simulink model "pr735_DDC_demodulation"  (R2018b)
settings: Solver=VariableStepAuto  StartTime=0.0  StopTime=2048/fs  RelTol=1e-3
PreLoadFcn:
  | fs=1e8;
  | pr731_DUC_setup
  | pr734_DDC_setup;
  | fc=40e6;
undefined symbols (not defined in the file or in its folder): CFIR, CIC, DCIC, designMultirateFIR, RRC
libraries: dspmlti4 x12, commdigbbndpm3 x2, commrandsrc3 x1
settings Model: Creator=Григорий Фокин  LastModifiedBy=Григорий Фокин
settings DataIOCC: SaveFormat=Array  SaveOutput=off  SignalLogging=off  SaveTime=off
settings DebuggingCC: AlgebraicLoopMsg=error
settings HardwareCC: ProdBitPerPointer=32  ProdBitPerSizeT=32  ProdBitPerPtrDiffT=32  ProdLargestAtomicFloat=None  ProdIntDivRoundTo=Undefined  ProdEndianess=Unspecified  ProdWordSize=32  ProdHWDeviceType=ASIC/FPGA->ASIC/FPGA  TargetBitPerPointer=64  TargetBitPerSizeT=64  TargetBitPerPtrDiffT=64  TargetLongLongMode=on  TargetIntDivRoundTo=Zero  TargetEndianess=LittleEndian  TargetWordSize=64  TargetHWDeviceType=Custom Processor->MATLAB Host Computer  ProdEqTarget=off

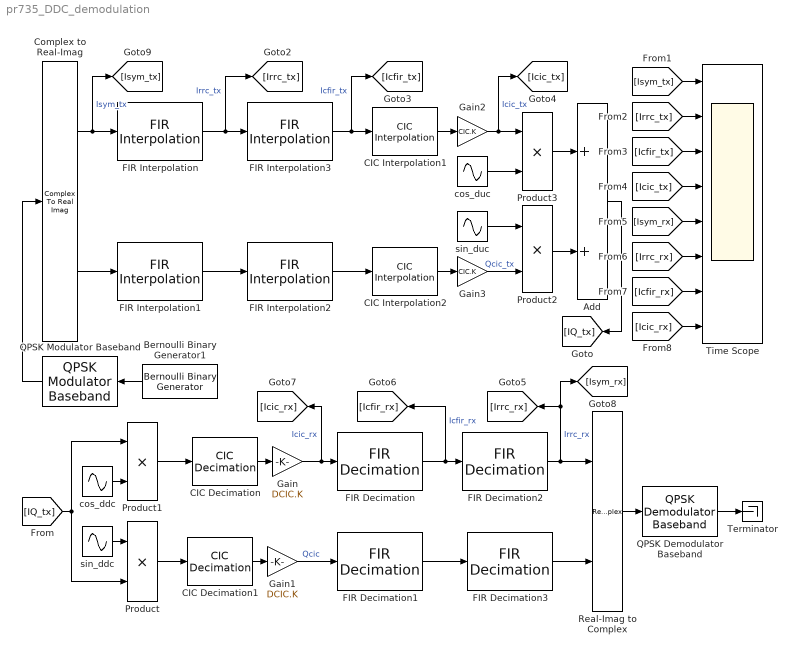
== system pr735_DDC_demodulation ==
  Add : Sum
  Bernoulli Binary Generator1 : commrandsrc3/Bernoulli Binary Generator  ProbabilityOfZero=0.5  SeedSource=Auto  Seed=0  SampleTime=(0.5*CIC.R*RRC.Lfactor*CFIR.Lfactor)/fs  SamplesPerFrame=2  OutputDataType=boolean  SimulateUsing=Interpreted execution
  CIC Decimation : dspmlti4/CIC Decimation  filtFrom=Multirate object in workspace  filtobj=hDCIC  ftype=Decimator  R=2  M=1  N=2  filterInternals=Full precision  BPS=[16 16 16 16]  FLPS=0  outputWordLength=32  outputFracLength=0  launchFVT=off  framing=Maintain input frame rate  RateOptions=Allow multirate processing
      settings: SourceProductName=DSP System Toolbox  SourceProductBaseCode=DS
  CIC Decimation1 : dspmlti4/CIC Decimation  filtFrom=Multirate object in workspace  filtobj=hDCIC  ftype=Decimator  R=2  M=1  N=2  filterInternals=Full precision  BPS=[16 16 16 16]  FLPS=0  outputWordLength=32  outputFracLength=0  launchFVT=off  framing=Maintain input frame rate  RateOptions=Allow multirate processing
      settings: SourceProductName=DSP System Toolbox  SourceProductBaseCode=DS
  CIC Interpolation1 : dspmlti4/CIC Interpolation  filtFrom=Multirate object in workspace  filtobj=hCIC  ftype=Interpolator  R=2  M=1  N=2  filterInternals=Full precision  BPS=[16 16 16 16]  FLPS=0  outputWordLength=32  outputFracLength=0  launchFVT=off  framing=Allow multirate processing  OutputFrames=off
      settings: SourceProductName=DSP System Toolbox  SourceProductBaseCode=DS
  CIC Interpolation2 : dspmlti4/CIC Interpolation  filtFrom=Multirate object in workspace  filtobj=hCIC  ftype=Interpolator  R=2  M=1  N=2  filterInternals=Full precision  BPS=[16 16 16 16]  FLPS=0  outputWordLength=32  outputFracLength=0  launchFVT=off  framing=Allow multirate processing  OutputFrames=off
      settings: SourceProductName=DSP System Toolbox  SourceProductBaseCode=DS
  Complex to Real-Imag : ComplexToRealImag
  FIR Decimation : dspmlti4/FIR Decimation  FilterSource=Filter object  h=designMultirateFIR(1,2)  D=2  filtStruct=Direct form  FilterObject=hDCFIR  framing=Enforce single-rate processing  inputOffset=0  outputBufInitCond=0  roundingMode=Floor  overflowMode=off  firstCoeffDataTypeStr=Inherit: Same word length as input  firstCoeffMin=[]  firstCoeffMax=[]  firstCoeffLastDataTypeStr=Inherit: Same word length as input  outputDataTypeStr=Inherit: Same as accumulator  outputMin=[]  outputMax=[]  outputLastDataTypeStr=Inherit: Same as accumulator
  FIR Decimation1 : dspmlti4/FIR Decimation  FilterSource=Filter object  h=designMultirateFIR(1,2)  D=2  filtStruct=Direct form  FilterObject=hDCFIR  framing=Enforce single-rate processing  inputOffset=0  outputBufInitCond=0  roundingMode=Floor  overflowMode=off  firstCoeffDataTypeStr=Inherit: Same word length as input  firstCoeffMin=[]  firstCoeffMax=[]  firstCoeffLastDataTypeStr=Inherit: Same word length as input  outputDataTypeStr=Inherit: Same as accumulator  outputMin=[]  outputMax=[]  outputLastDataTypeStr=Inherit: Same as accumulator
  FIR Decimation2 : dspmlti4/FIR Decimation  FilterSource=Filter object  h=designMultirateFIR(1,2)  D=2  filtStruct=Direct form  FilterObject=hDRRC  framing=Enforce single-rate processing  inputOffset=0  outputBufInitCond=0  roundingMode=Floor  overflowMode=off  firstCoeffDataTypeStr=Inherit: Same word length as input  firstCoeffMin=[]  firstCoeffMax=[]  firstCoeffLastDataTypeStr=Inherit: Same word length as input  outputDataTypeStr=Inherit: Same as accumulator  outputMin=[]  outputMax=[]  outputLastDataTypeStr=Inherit: Same as accumulator
  FIR Decimation3 : dspmlti4/FIR Decimation  FilterSource=Filter object  h=designMultirateFIR(1,2)  D=2  filtStruct=Direct form  FilterObject=hDRRC  framing=Enforce single-rate processing  inputOffset=0  outputBufInitCond=0  roundingMode=Floor  overflowMode=off  firstCoeffDataTypeStr=Inherit: Same word length as input  firstCoeffMin=[]  firstCoeffMax=[]  firstCoeffLastDataTypeStr=Inherit: Same word length as input  outputDataTypeStr=Inherit: Same as accumulator  outputMin=[]  outputMax=[]  outputLastDataTypeStr=Inherit: Same as accumulator
  FIR Interpolation : dspmlti4/FIR Interpolation  FilterSource=Filter object  h=designMultirateFIR(3,1)  L=3  FilterObject=hRRC  framing=Enforce single-rate processing  outputBufInitCond=0  roundingMode=Floor  overflowMode=off  firstCoeffDataTypeStr=Inherit: Same word length as input  firstCoeffMin=[]  firstCoeffMax=[]  firstCoeffLastDataTypeStr=Inherit: Same word length as input  outputDataTypeStr=Inherit: Same as accumulator  outputMin=[]  outputMax=[]  outputLastDataTypeStr=Inherit: Same as accumulator
      settings: SourceProductName=DSP System Toolbox
  FIR Interpolation1 : dspmlti4/FIR Interpolation  FilterSource=Filter object  h=designMultirateFIR(3,1)  L=3  FilterObject=hRRC  framing=Enforce single-rate processing  outputBufInitCond=0  roundingMode=Floor  overflowMode=off  firstCoeffDataTypeStr=Inherit: Same word length as input  firstCoeffMin=[]  firstCoeffMax=[]  firstCoeffLastDataTypeStr=Inherit: Same word length as input  outputDataTypeStr=Inherit: Same as accumulator  outputMin=[]  outputMax=[]  outputLastDataTypeStr=Inherit: Same as accumulator
      settings: SourceProductName=DSP System Toolbox
  FIR Interpolation2 : dspmlti4/FIR Interpolation  FilterSource=Filter object  h=designMultirateFIR(3,1)  L=3  FilterObject=hCFIR  framing=Enforce single-rate processing  outputBufInitCond=0  roundingMode=Floor  overflowMode=off  firstCoeffDataTypeStr=Inherit: Same word length as input  firstCoeffMin=[]  firstCoeffMax=[]  firstCoeffLastDataTypeStr=Inherit: Same word length as input  outputDataTypeStr=Inherit: Same as accumulator  outputMin=[]  outputMax=[]  outputLastDataTypeStr=Inherit: Same as accumulator
      settings: SourceProductName=DSP System Toolbox
  FIR Interpolation3 : dspmlti4/FIR Interpolation  FilterSource=Filter object  h=designMultirateFIR(3,1)  L=3  FilterObject=hCFIR  framing=Enforce single-rate processing  outputBufInitCond=0  roundingMode=Floor  overflowMode=off  firstCoeffDataTypeStr=Inherit: Same word length as input  firstCoeffMin=[]  firstCoeffMax=[]  firstCoeffLastDataTypeStr=Inherit: Same word length as input  outputDataTypeStr=Inherit: Same as accumulator  outputMin=[]  outputMax=[]  outputLastDataTypeStr=Inherit: Same as accumulator
      settings: SourceProductName=DSP System Toolbox
  Gain : Gain  Gain=DCIC.K  OutMin=-1  OutMax=1  OutDataTypeStr=fixdt(1,16)
  Gain1 : Gain  Gain=DCIC.K  OutMin=-1  OutMax=1  OutDataTypeStr=fixdt(1,16)
  Gain2 : Gain  Gain=CIC.K  OutMin=-1  OutMax=1  OutDataTypeStr=fixdt(1,16)
  Gain3 : Gain  Gain=CIC.K  OutMin=-1  OutMax=1  OutDataTypeStr=fixdt(1,16)
  Product : Product  OutMin=-1  OutMax=-1  OutDataTypeStr=fixdt(1,16)
  Product1 : Product  OutMin=-1  OutMax=1  OutDataTypeStr=fixdt(1,16)
  Product2 : Product
  Product3 : Product
  QPSK Demodulator Baseband : commdigbbndpm3/QPSK Demodulator Baseband  OutType=Bit  DecType=Hard decision  VarSource=Dialog  Variance=1  Dec=Gray  Ph=pi/4  outDtype1=boolean  outDtype2=Inherit via internal rule  derotateFactorWordLen=16  derotateFactorDataTypeStr=Inherit: Same word length as input  derotateFactorLastDataTypeStr=Inherit: Same word length as input
  QPSK Modulator Baseband : commdigbbndpm3/QPSK Modulator Baseband  InType=Bit  Enc=Gray  Ph=pi/4  outDtype=Fixed-point  outWordLen=16  outUDDataType=sfix(16)  outFracLenMode=Best precision  outFracLen=15  outDataTypeStr=fixdt(1,16)  outLastDataTypeStr=fixdt(1,16)
  Real-Imag to Complex : RealImagToComplex
  Terminator : Terminator
  Time Scope : Scope  NumInputPorts=8
  cos_ddc : Sin  Frequency=fc*2*pi  Phase=pi/2  SampleTime=1/fs
  cos_duc : Sin  Frequency=fc*2*pi  Phase=pi/2  SampleTime=1/fs
  sin_ddc : Sin  Frequency=fc*2*pi  SampleTime=1/fs
  sin_duc : Sin  Frequency=fc*2*pi  SampleTime=1/fs
  wires:
  cos_ddc/1 -> Product1/2
  sin_ddc/1 -> Product/1
  [IQ_tx] -> Product/2, Product1/1
  Product1/1 -> CIC Decimation/1
  Product/1 -> CIC Decimation1/1
  CIC Decimation/1 -> Gain/1
  CIC Decimation1/1 -> Gain1/1
  Gain/1 -> [Icic_rx], FIR Decimation/1  "Icic_rx"
  Gain1/1 -> FIR Decimation1/1  "Qcic"
  FIR Decimation/1 -> FIR Decimation2/1, [Icfir_rx]  "Icfir_rx"
  FIR Decimation1/1 -> FIR Decimation3/1
  FIR Decimation2/1 -> Real-Imag to Complex/1, [Isym_rx], [Irrc_rx]  "Irrc_rx"
  Real-Imag to Complex/1 -> QPSK Demodulator Baseband/1
  FIR Interpolation1/1 -> FIR Interpolation2/1
  FIR Interpolation/1 -> FIR Interpolation3/1, [Irrc_tx]  "Irrc_tx"
  cos_duc/1 -> Product3/2
  Add/1 -> [IQ_tx]
  Complex to Real-Imag/1 -> [Isym_tx], FIR Interpolation/1  "Isym_tx"
  Product2/1 -> Add/2
  Gain2/1 -> Product3/1, [Icic_tx]  "Icic_tx"
  Product3/1 -> Add/1
  Gain3/1 -> Product2/2  "Qcic_tx"
  QPSK Modulator Baseband/1 -> Complex to Real-Imag/1
  FIR Interpolation2/1 -> CIC Interpolation2/1
  Complex to Real-Imag/2 -> FIR Interpolation1/1
  Bernoulli Binary Generator1/1 -> QPSK Modulator Baseband/1
  sin_duc/1 -> Product2/1
  FIR Interpolation3/1 -> CIC Interpolation1/1, [Icfir_tx]  "Icfir_tx"
  CIC Interpolation1/1 -> Gain2/1
  CIC Interpolation2/1 -> Gain3/1
  [Isym_tx] -> Time Scope/1
  [Irrc_tx] -> Time Scope/2
  [Icfir_tx] -> Time Scope/3
  [Icic_tx] -> Time Scope/4
  [Isym_rx] -> Time Scope/5
  [Irrc_rx] -> Time Scope/6
  [Icfir_rx] -> Time Scope/7
  [Icic_rx] -> Time Scope/8
  FIR Decimation3/1 -> Real-Imag to Complex/2
  QPSK Demodulator Baseband/1 -> Terminator/1
